simulink model "LATC_Test_Calc"  (R2021b)
settings: Solver=FixedStepDiscrete  StartTime=0.0  StopTime=inf  FixedStep=0.01  RelTol=1e-3
undefined symbols (not defined in the file or in its folder): P_LCS_A0_Dis_BP, P_LCS_A2_Curve_BP, P_LCS_A2S_FliterTime, P_LCS_DeltaEps_SpdBp, P_LCS_LCC_A0_Dis_BP, P_LCS_LCC_AngleSlope_ELK, P_LCS_LCC_AngleSlope_ESS, P_LCS_LCC_AngleSlope_LCCancle, P_LCS_LCC_AngleSlope_LCEco, P_LCS_LCC_AngleSlope_LCK, P_LCS_LCC_AngleSlope_LCKIE, P_LCS_LCC_AngleSlope_LCNomal, P_LCS_LCC_AngleSlope_LCSport, P_LCS_LCC_AngleSlope_LKA, P_LCS_LCC_Eco_AyDtLimit_TBL, P_LCS_LCC_ELK_AyDtLimit_TBL, P_LCS_LCC_ESS_AyDtLimit_TBL, P_LCS_LCC_LC_AyDtLimit_TBL, P_LCS_LCC_LC_Normal_AyDtLimit_TBL, P_LCS_LCC_LC_Planning_Dist_TBL, P_LCS_LCC_LCK_AyDtLimit_TBL, P_LCS_LCC_LCK_Planning_Dist_TBL, P_LCS_LCC_LKA_AyDtLimit_TBL, P_LCS_LCC_Matrix_q1_st, P_LCS_LCC_Matrix_q2_st, P_LCS_LCC_Max_Lateral_Acc_ms2, P_LCS_LCC_MaxLatAcc_ELK, P_LCS_LCC_MaxLatAcc_ESS, P_LCS_LCC_MaxLatAcc_LCCancel, P_LCS_LCC_MaxLatAcc_LCEco, P_LCS_LCC_MaxLatAcc_LCK, P_LCS_LCC_MaxLatAcc_LCKIE, P_LCS_LCC_MaxLatAcc_LCNomal, P_LCS_LCC_MaxLatAcc_LCSport, P_LCS_LCC_MaxLatAcc_LKA, P_LCS_LCC_Min_Plan_Dis, P_LCS_LCC_PlaningLength_m, P_LCS_LCC_PreCur_Min_Plan_Dis_Fac, P_LCS_LCC_PreView_Fac, P_LCS_LCC_PreView_s, P_LCS_LCC_PreViewCurve_Fac, P_LCS_LCC_PreViewT, P_LCS_LCC_Spd_BP, P_LCS_LCC_Spd_BP2, P_LCS_LCC_Sport_AyDtLimit_TBL, P_LCS_LCC_StateActiv_AyDtLimit, P_LCS_LCC_StateActiv_PreviewT, P_LCS_LCC_StateActiveDelaytime, P_LCS_LCC_TarSteerAngleSlope, P_LCS_preDis_spd, P_LCS_StateActiv_AngleSlope, P_LCS_StateActive_HoldTime_BP, P_LCS_StateActiveFlg_BP, P_LCS_StateHold_time
libraries: canapelib x35, simulink x2
(part 1 of 3)
settings Model: DataDictionary=HWAtest.sldd  Creator=GW00216231  LastModifiedBy=GW00201118
settings SolverCC: AlgebraicLoopSolver=TrustRegion
settings OptimizationCC: DefaultParameterBehavior=Inlined  EnhancedBackFolding=on  PassReuseOutputArgsThreshold=0  OptimizeBlockOrder=speed  DifferentSizesBufferReuse=on  OptimizationCustomize=off
settings DebuggingCC: SignalResolutionControl=TryResolveAllWithWarning  ParameterTunabilityLossMsg=error  SFMachineParentedDataDiag=warning  UnderSpecifiedDimensionMsg=warning
settings SFSimCC: MATLABDynamicMemAlloc=off
settings RTWCC: Description=Vector CANape/vSignalyzer Target (Visual C/C++ Project Makefile)  SystemTargetFile=cnp.tlc  TemplateMakefile=cnp_msdll.tmf
settings CodeAppCC: ForceParamTrailComments=on  OperatorAnnotations=on
settings STFCustomTargetCC: MATLABClassNameForMDSCustomization=Simulink.SoftwareTarget.TargetSpecificTriggerConfigurationBase  SystemTargetFile=cnp.tlc

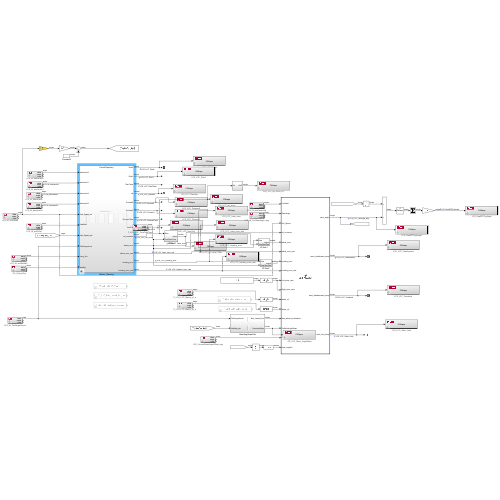
[thumbnail: Simulink's stored preview of the top-level diagram]
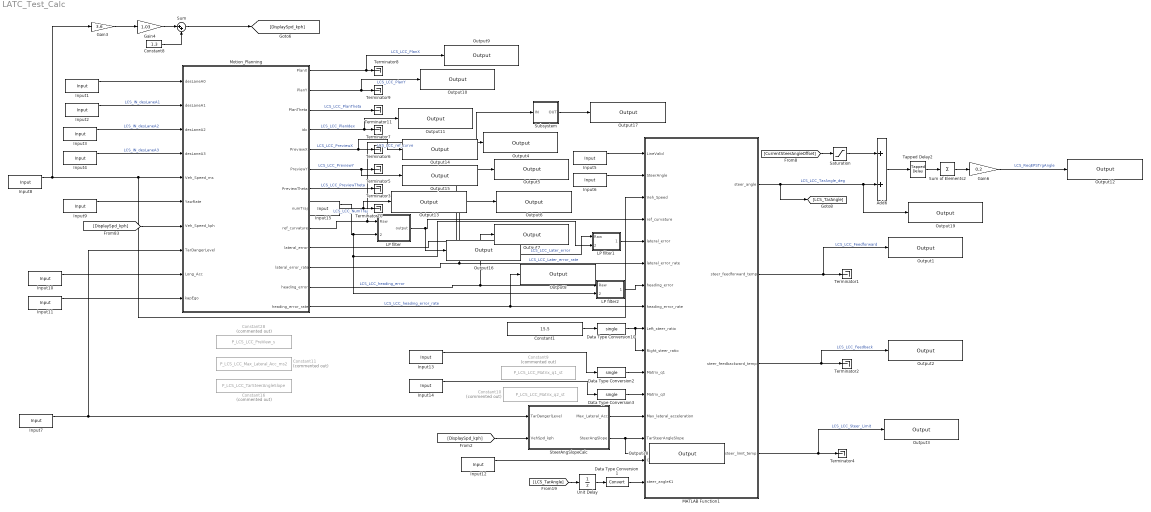
== system LATC_Test_Calc ==
  Add6 : Sum  AccumDataTypeStr=single
  Constant1 : Constant  Value=15.5  OutDataTypeStr=single
  Constant10 : Constant  Commented=on  Value=P_LCS_LCC_Matrix_q2_st  OutDataTypeStr=single
  Constant11 : Constant  Commented=on  Value=P_LCS_LCC_Max_Lateral_Acc_ms2  OutDataTypeStr=single
  Constant16 : Constant  Commented=on  Value=P_LCS_LCC_TarSteerAngleSlope  OutDataTypeStr=single
  Constant28 : Constant  Commented=on  Value=P_LCS_LCC_PreView_s  OutDataTypeStr=single
  Constant8 : Constant  Value=1.3  OutDataTypeStr=single
  Constant9 : Constant  Commented=on  Value=P_LCS_LCC_Matrix_q1_st  OutDataTypeStr=single
  Data Type Conversion1 : DataTypeConversion
  Data Type Conversion10 : DataTypeConversion  OutDataTypeStr=single
  Data Type Conversion2 : DataTypeConversion  OutDataTypeStr=single
  Data Type Conversion3 : DataTypeConversion  OutDataTypeStr=single
  Gain3 : Gain  Gain=3.6
  Gain4 : Gain  Gain=1.03
  Gain6 : Gain  Gain=0.2
  Input1 : canapelib/CANape I//O/Input  envName=LCS_IN_desLaneA0  envRows=1  envCols=1  envDataType=float  swInheritSampleTime=on  envPortId=0
      settings: AttributesFormatString=%<envName>  SourceProductName=Vector CANape/vSignalyzer Target
  Input10 : canapelib/CANape I//O/Input  envName=LCS_IN_axvRefMs2  envRows=1  envCols=1  envDataType=float  swInheritSampleTime=on  envPortId=0
      settings: AttributesFormatString=%<envName>  SourceProductName=Vector CANape/vSignalyzer Target
  Input11 : canapelib/CANape I//O/Input  envName=LCS_IN_kapTraj  envRows=1  envCols=1  envDataType=float  swInheritSampleTime=on  envPortId=0
      settings: AttributesFormatString=%<envName>  SourceProductName=Vector CANape/vSignalyzer Target
  Input12 : canapelib/CANape I//O/Input  envName=LCS_CurrentSteerAngleOffset_deg  envRows=1  envCols=1  envDataType=float  swInheritSampleTime=on  envPortId=0
      settings: AttributesFormatString=%<envName>  SourceProductName=Vector CANape/vSignalyzer Target
  Input13 : canapelib/CANape I//O/Input  envName=P_LCS_LCC_Matrix_q1_st  envRows=1  envCols=1  envDataType=float  swInheritSampleTime=on  envPortId=0
      settings: AttributesFormatString=%<envName>  SourceProductName=Vector CANape/vSignalyzer Target
  Input14 : canapelib/CANape I//O/Input  envName=P_LCS_LCC_Matrix_q2_st  envRows=1  envCols=1  envDataType=float  swInheritSampleTime=on  envPortId=0
      settings: AttributesFormatString=%<envName>  SourceProductName=Vector CANape/vSignalyzer Target
  Input15 : canapelib/CANape I//O/Input  envName=P_LCS_LCC_CureFilterTime  envRows=1  envCols=1  envDataType=float  swInheritSampleTime=on  envPortId=0
      settings: AttributesFormatString=%<envName>  SourceProductName=Vector CANape/vSignalyzer Target
  Input2 : canapelib/CANape I//O/Input  envName=LCS_IN_desLaneA1  envRows=1  envCols=1  envDataType=float  swInheritSampleTime=on  envPortId=0
      settings: AttributesFormatString=%<envName>  SourceProductName=Vector CANape/vSignalyzer Target
  Input3 : canapelib/CANape I//O/Input  envName=LCS_IN_desLaneA2  envRows=1  envCols=1  envDataType=float  swInheritSampleTime=on  envPortId=0
      settings: AttributesFormatString=%<envName>  SourceProductName=Vector CANape/vSignalyzer Target
  Input4 : canapelib/CANape I//O/Input  envName=LCS_IN_desLaneA3  envRows=1  envCols=1  envDataType=float  swInheritSampleTime=on  envPortId=0
      settings: AttributesFormatString=%<envName>  SourceProductName=Vector CANape/vSignalyzer Target
  Input5 : canapelib/CANape I//O/Input  envName=LCS_IN_desLaneValid  envRows=1  envCols=1  envDataType=float  swInheritSampleTime=on  envPortId=0
      settings: AttributesFormatString=%<envName>  SourceProductName=Vector CANape/vSignalyzer Target
  Input6 : canapelib/CANape I//O/Input  envName=LCS_IN_CurSteerAngle_deg  envRows=1  envCols=1  envDataType=float  swInheritSampleTime=on  envPortId=0
      settings: AttributesFormatString=%<envName>  SourceProductName=Vector CANape/vSignalyzer Target
  Input7 : canapelib/CANape I//O/Input  envName=LCS_IN_TarDangerlLevel  envRows=1  envCols=1  envDataType=uint8  swInheritSampleTime=on  envPortId=0
      settings: AttributesFormatString=%<envName>  SourceProductName=Vector CANape/vSignalyzer Target
  Input8 : canapelib/CANape I//O/Input  envName=LCS_IN_vxvRefMs  envRows=1  envCols=1  envDataType=float  swInheritSampleTime=on  envPortId=0
      settings: AttributesFormatString=%<envName>  SourceProductName=Vector CANape/vSignalyzer Target
  Input9 : canapelib/CANape I//O/Input  envName=LCS_IN_psiDtOpt  envRows=1  envCols=1  envDataType=float  swInheritSampleTime=on  envPortId=0
      settings: AttributesFormatString=%<envName>  SourceProductName=Vector CANape/vSignalyzer Target
  LP filter : Subsystem
  LP filter1 : Subsystem
  LP filter2 : Subsystem
  MATLAB Function1 : MATLAB Function  TreatAsAtomicUnit=on
  Motion_Planning : Subsystem  Variant=on  VariantControlMode=label  LabelModeActiveChoice=Choice_3
  Output1 : canapelib/CANape I//O/Output  envName=LCS_LCC_Feedforward  envRows=1  envCols=1  envPortId=0
      settings: AttributesFormatString=%<envName>  SourceProductName=Vector CANape/vSignalyzer Target
  Output10 : canapelib/CANape I//O/Output  envName=LCS_LCC_PlanY  envRows=40  envCols=1  envPortId=0
      settings: AttributesFormatString=%<envName>  SourceProductName=Vector CANape/vSignalyzer Target
  Output11 : canapelib/CANape I//O/Output  envName=LCS_LCC_PlanIdex  envRows=1  envCols=1  envPortId=0
      settings: AttributesFormatString=%<envName>  SourceProductName=Vector CANape/vSignalyzer Target
  Output12 : canapelib/CANape I//O/Output  envName=LCS_ReqEPSTrgAngle  envRows=1  envCols=1  envPortId=0
      settings: AttributesFormatString=%<envName>  SourceProductName=Vector CANape/vSignalyzer Target
  Output13 : canapelib/CANape I//O/Output  envName=LCS_LCC_NumTraj  envRows=1  envCols=1  envPortId=0
      settings: AttributesFormatString=%<envName>  SourceProductName=Vector CANape/vSignalyzer Target
  Output14 : canapelib/CANape I//O/Output  envName=LCS_LCC_PreviewX  envRows=1  envCols=1  envPortId=0
      settings: AttributesFormatString=%<envName>  SourceProductName=Vector CANape/vSignalyzer Target
  Output15 : canapelib/CANape I//O/Output  envName=LCS_LCC_PreviewY  envRows=1  envCols=1  envPortId=0
      settings: AttributesFormatString=%<envName>  SourceProductName=Vector CANape/vSignalyzer Target
  Output16 : canapelib/CANape I//O/Output  envName=LCS_LCC_ref_curve_Filter  envRows=1  envCols=1  envPortId=0
      settings: AttributesFormatString=%<envName>  SourceProductName=Vector CANape/vSignalyzer Target
  Output17 : canapelib/CANape I//O/Output  envName=LCS_LCC_ref_curve_Av  envRows=1  envCols=1  envPortId=0
      settings: AttributesFormatString=%<envName>  SourceProductName=Vector CANape/vSignalyzer Target
  Output18 : canapelib/CANape I//O/Output  envName=LCS_LCC_Steer_AngleSlope  envRows=1  envCols=1  envPortId=0
      settings: AttributesFormatString=%<envName>  SourceProductName=Vector CANape/vSignalyzer Target
  Output19 : canapelib/CANape I//O/Output  envName=LCS_ReqEPSTrgAngle1  envRows=1  envCols=1  envPortId=0
      settings: AttributesFormatString=%<envName>  SourceProductName=Vector CANape/vSignalyzer Target
  Output2 : canapelib/CANape I//O/Output  envName=LCS_LCC_Feedback  envRows=1  envCols=1  envPortId=0
      settings: AttributesFormatString=%<envName>  SourceProductName=Vector CANape/vSignalyzer Target
  Output3 : canapelib/CANape I//O/Output  envName=LCS_LCC_Steer_Limit  envRows=1  envCols=1  envPortId=0
      settings: AttributesFormatString=%<envName>  SourceProductName=Vector CANape/vSignalyzer Target
  Output4 : canapelib/CANape I//O/Output  envName=LCS_LCC_ref_curve  envRows=1  envCols=1  envPortId=0
      settings: AttributesFormatString=%<envName>  SourceProductName=Vector CANape/vSignalyzer Target
  Output5 : canapelib/CANape I//O/Output  envName=LCS_LCC_Later_error  envRows=1  envCols=1  envPortId=0
      settings: AttributesFormatString=%<envName>  SourceProductName=Vector CANape/vSignalyzer Target
  Output6 : canapelib/CANape I//O/Output  envName=LCS_LCC_Later_error_rate  envRows=1  envCols=1  envPortId=0
      settings: AttributesFormatString=%<envName>  SourceProductName=Vector CANape/vSignalyzer Target
  Output7 : canapelib/CANape I//O/Output  envName=LCS_LCC_heading_error  envRows=1  envCols=1  envPortId=0
      settings: AttributesFormatString=%<envName>  SourceProductName=Vector CANape/vSignalyzer Target
  Output8 : canapelib/CANape I//O/Output  envName=LCS_LCC_heading_error_rate  envRows=1  envCols=1  envPortId=0
      settings: AttributesFormatString=%<envName>  SourceProductName=Vector CANape/vSignalyzer Target
  Output9 : canapelib/CANape I//O/Output  envName=LCS_LCC_PlanX  envRows=40  envCols=1  envPortId=0
      settings: AttributesFormatString=%<envName>  SourceProductName=Vector CANape/vSignalyzer Target
  Saturation : Saturate  UpperLimit=10  LowerLimit=-10  OutDataTypeStr=single
  SteerAngSlopeCalc : Subsystem
  Subsystem : Subsystem
  Sum : Sum  Inputs=|++
  Sum of Elements2 : Sum  Inputs=+
  Tapped Delay2 : simulink/Discrete/Tapped Delay  vinit=0.0  samptime=-1  NumDelays=4  DelayOrder=Newest  includeCurrent=on
  Terminator{1..11} (11 alike) : Terminator
  Unit Delay : UnitDelay  SampleTime=-1  HasFrameUpgradeWarning=on
  wires:
  [DisplaySpd_kph] -> Motion_Planning/7(Veh_Speed_kph)
  Input10/1 -> Motion_Planning/9(Long_Acc)
  Sum of Elements2/1 -> Gain6/1
  Motion_Planning/11(lateral_error_rate) -> Output6/1, MATLAB Function1/6(lateral_error_rate)  "LCS_LCC_Later_error_rate"
  Input8/1 -> Gain3/1, MATLAB Function1/3(Veh_Speed), Motion_Planning/5(Veh_Speed_ms)
  MATLAB Function1/2(steer_feedforward_temp) -> Output1/1, Terminator1/1  "LCS_LCC_Feedforward"
  Input12/1 -> MATLAB Function1/15(CurrentSteerAngleOffset)
  Gain6/1 -> Output12/1  "LCS_ReqEPSTrgAngle"
  MATLAB Function1/4(steer_limit_temp) -> Output3/1, Terminator4/1  "LCS_LCC_Steer_Limit"
  SteerAngSlopeCalc/1(Max_Lateral_Acc) -> MATLAB Function1/13(Max_lateral_acceleration)
  Add6/1 -> Tapped Delay2/1
  SteerAngSlopeCalc/2(SteerAngSlope) -> Output18/1, MATLAB Function1/14(TarSteerAngleSlope)
  [LCS_TarAngle] -> Unit Delay/1
  MATLAB Function1/3(steer_feedbackward_temp) -> Output2/1, Terminator2/1  "LCS_LCC_Feedback"
  Motion_Planning/4(idx) -> Output11/1, Terminator7/1  "LCS_LCC_PlanIdex"
  [DisplaySpd_kph] -> SteerAngSlopeCalc/2(VehSpd_kph)
  LP filter/1(output) -> Output16/1, MATLAB Function1/4(ref_curvature)
  Data Type Conversion2/1 -> MATLAB Function1/11(Matrix_q1)
  Motion_Planning/10(lateral_error) -> LP filter1/1(Raw), Output5/1  "LCS_LCC_Later_error"
  Motion_Planning/2(PlanY) -> Output10/1, Terminator9/1  "LCS_LCC_PlanY"
  Motion_Planning/6(PreviewY) -> Output15/1, Terminator5/1  "LCS_LCC_PreviewY"
  Input5/1 -> MATLAB Function1/1(LineValid)
  Input1/1 -> Motion_Planning/1(desLaneA0)
  Saturation/1 -> Add6/1
  Input6/1 -> MATLAB Function1/2(SteerAngle)
  Motion_Planning/3(PlanTheta) -> Terminator11/1  "LCS_LCC_PlanTheta"
  Motion_Planning/12(heading_error) -> Output7/1, LP filter2/1(Raw)  "LCS_LCC_heading_error"
  Unit Delay/1 -> Data Type Conversion1/1
  Input2/1 -> Motion_Planning/2(desLaneA1)  "LCS_IN_desLaneA1"
  Input11/1 -> Motion_Planning/10(kapEgo)
  Data Type Conversion10/1 -> MATLAB Function1/10(Right_steer_ratio), MATLAB Function1/9(Left_steer_ratio)
  Input14/1 -> Data Type Conversion3/1
  Input4/1 -> Motion_Planning/4(desLaneA3)  "LCS_IN_desLaneA3"
  Motion_Planning/7(PreviewTheta) -> Terminator3/1  "LCS_LCC_PreviewTheta"
  Input7/1 -> Motion_Planning/8(TarDangerLevel), SteerAngSlopeCalc/1(TarDangerlLevel)
  Motion_Planning/13(heading_error_rate) -> Output8/1, MATLAB Function1/8(heading_error_rate)  "LCS_LCC_heading_error_rate"
  Tapped Delay2/1 -> Sum of Elements2/1
  Input9/1 -> Motion_Planning/6(YawRate)
  Input3/1 -> Motion_Planning/3(desLaneA2)  "LCS_IN_desLaneA2"
  Data Type Conversion1/1 -> MATLAB Function1/16(steer_angleK1)
  [CurrentSteerAngleOffset] -> Saturation/1
  MATLAB Function1/1(steer_angle) -> [LCS_TarAngle], Output19/1, Add6/2  "LCS_LCC_TarAngle_deg"
  Motion_Planning/1(PlanX) -> Output9/1, Terminator8/1  "LCS_LCC_PlanX"
  Constant1/1 -> Data Type Conversion10/1
  Motion_Planning/5(PreviewX) -> Output14/1, Terminator6/1  "LCS_LCC_PreviewX"
  Data Type Conversion3/1 -> MATLAB Function1/12(Matrix_q3)
  Motion_Planning/8(numTraj) -> Output13/1, Terminator10/1  "LCS_LCC_NumTraj"
  Input13/1 -> Data Type Conversion2/1
  Sum/1 -> [DisplaySpd_kph]
  Gain3/1 -> Gain4/1
  Gain4/1 -> Sum/1
  Constant8/1 -> Sum/2
  Motion_Planning/9(ref_curvature) -> Subsystem/1(IN), Output4/1, LP filter/1(Raw)  "LCS_LCC_ref_curve"
  Subsystem/1(OUT) -> Output17/1
  LP filter1/1(output) -> MATLAB Function1/5(lateral_error)
  LP filter2/1(output) -> MATLAB Function1/7(heading_error)
  Input15/1 -> LP filter2/2(TorqFilterTime), LP filter1/2(TorqFilterTime), LP filter/2(TorqFilterTime)

== system LATC_Test_Calc/LP filter ==
  Raw : Inport
  TorqFilterTime : Inport  Port=2
  Memory2 : Memory  InheritSampleTime=on
  Product1 : Product  RndMeth=Zero
  Product4 : Product  Inputs=*/  RndMeth=Zero
  Sum4 : Sum  Inputs=+-|
  Sum5 : Sum  Inputs=++|
  Weight/N3 : Constant  Value=0.02  OutDataTypeStr=single
  output : Outport
  wires:
  TorqFilterTime/1 -> Product4/2
  Product4/1 -> Product1/1
  Weight/N3/1 -> Product4/1
  Raw/1 -> Sum4/1
  Product1/1 -> Sum5/1
  Sum4/1 -> Product1/2
  Memory2/1 -> Sum4/2, Sum5/2
  Sum5/1 -> output/1, Memory2/1

== system LATC_Test_Calc/LP filter1 ==
  Raw : Inport
  TorqFilterTime : Inport  Port=2
  Memory2 : Memory  InheritSampleTime=on
  Product1 : Product  RndMeth=Zero
  Product4 : Product  Inputs=*/  RndMeth=Zero
  Sum4 : Sum  Inputs=+-|
  Sum5 : Sum  Inputs=++|
  Weight/N3 : Constant  Value=0.02  OutDataTypeStr=single
  output : Outport
  wires:
  Sum5/1 -> Memory2/1, output/1
  Memory2/1 -> Sum5/2, Sum4/2
  Sum4/1 -> Product1/2
  Product1/1 -> Sum5/1
  Raw/1 -> Sum4/1
  Weight/N3/1 -> Product4/1
  Product4/1 -> Product1/1
  TorqFilterTime/1 -> Product4/2

== system LATC_Test_Calc/LP filter2 ==
  Raw : Inport
  TorqFilterTime : Inport  Port=2
  Memory2 : Memory  InheritSampleTime=on
  Product1 : Product  RndMeth=Zero
  Product4 : Product  Inputs=*/  RndMeth=Zero
  Sum4 : Sum  Inputs=+-|
  Sum5 : Sum  Inputs=++|
  Weight/N3 : Constant  Value=0.02  OutDataTypeStr=single
  output : Outport
  wires:
  TorqFilterTime/1 -> Product4/2
  Product4/1 -> Product1/1
  Weight/N3/1 -> Product4/1
  Raw/1 -> Sum4/1
  Product1/1 -> Sum5/1
  Sum4/1 -> Product1/2
  Memory2/1 -> Sum4/2, Sum5/2
  Sum5/1 -> output/1, Memory2/1

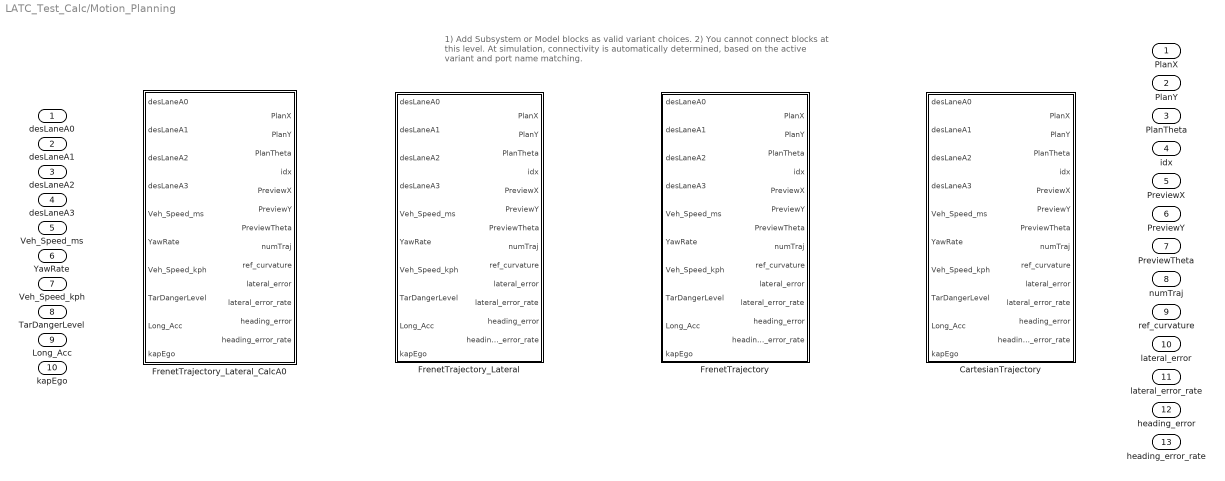
== system LATC_Test_Calc/Motion_Planning ==
  note: 1) Add Subsystem or Model blocks as valid variant choices.
      | 2) You cannot connect blocks at this level. At simulation, connectivity is automatically
      | determined, based on the active variant and port name matching.
  desLaneA0 : Inport
  desLaneA1 : Inport  Port=2
  desLaneA2 : Inport  Port=3
  desLaneA3 : Inport  Port=4
  Veh_Speed_ms : Inport  Port=5
  YawRate : Inport  Port=6
  Veh_Speed_kph : Inport  Port=7
  TarDangerLevel : Inport  Port=8
  Long_Acc : Inport  Port=9
  kapEgo : Inport  Port=10
  CartesianTrajectory : Subsystem  VariantControl=Choice_4
  FrenetTrajectory : Subsystem  VariantControl=Choice_3
  FrenetTrajectory_Lateral : Subsystem  VariantControl=Choice_2
  FrenetTrajectory_Lateral_CalcA0 : Subsystem  VariantControl=Choice_1
  PlanX : Outport
  PlanY : Outport  Port=2
  PlanTheta : Outport  Port=3
  idx : Outport  Port=4
  PreviewX : Outport  Port=5
  PreviewY : Outport  Port=6
  PreviewTheta : Outport  Port=7
  numTraj : Outport  Port=8
  ref_curvature : Outport  Port=9
  lateral_error : Outport  Port=10
  lateral_error_rate : Outport  Port=11
  heading_error : Outport  Port=12
  heading_error_rate : Outport  Port=13

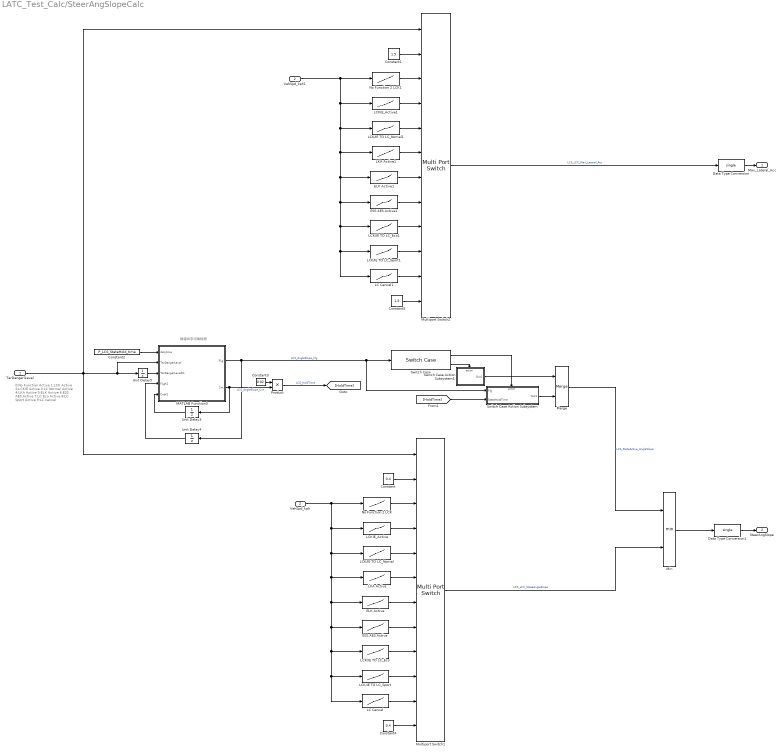
== system LATC_Test_Calc/SteerAngSlopeCalc ==
  note: 0:No Function Active
      | 1:LCK Active
      | 2:LCKIE Active
      | 3:LC Normal Active
      | 4:LKA Active
      | 5:ELK Active
      | 6:ESS AES Active
      | 7:LC Eco Active
      | 8:LC Sport Active
      | 9:LC cancel
  note: 换道状态切换检测
  TarDangerlLevel : Inport
  VehSpd_kph : Inport  Port=2
  Constant : Constant  Value=0.4  OutDataTypeStr=single
  Constant1 : Constant  Value=1.5  OutDataTypeStr=single
  Constant2 : Constant  Value=P_LCS_StateHold_time  OutDataTypeStr=uint16
  Constant3 : Constant  Value=0.02
  Constant4 : Constant  Value=0.4  OutDataTypeStr=single
  Constant5 : Constant  Value=1.5  OutDataTypeStr=single
  Data Type Conversion : DataTypeConversion  OutDataTypeStr=single
  Data Type Conversion1 : DataTypeConversion  OutDataTypeStr=single
  ELK Active : Lookup_n-D  NumberOfTableDimensions=1  BreakpointsForDimension1=P_LCS_preDis_spd  Table=P_LCS_LCC_AngleSlope_ELK  ExtrapMethod=Clip  InternalRulePriority=Speed  RndMeth=Simplest  InputSameDT=on
  ELK Active1 : Lookup_n-D  NumberOfTableDimensions=1  BreakpointsForDimension1=P_LCS_preDis_spd  Table=P_LCS_LCC_MaxLatAcc_ELK  ExtrapMethod=Clip  InternalRulePriority=Speed  RndMeth=Simplest  InputSameDT=on
  ESS AES Active : Lookup_n-D  NumberOfTableDimensions=1  BreakpointsForDimension1=P_LCS_preDis_spd  Table=P_LCS_LCC_AngleSlope_ESS  ExtrapMethod=Clip  InternalRulePriority=Speed  RndMeth=Simplest  InputSameDT=on
  ESS AES Active1 : Lookup_n-D  NumberOfTableDimensions=1  BreakpointsForDimension1=P_LCS_preDis_spd  Table=P_LCS_LCC_MaxLatAcc_ESS  ExtrapMethod=Clip  InternalRulePriority=Speed  RndMeth=Simplest  InputSameDT=on
  LC Cancel : Lookup_n-D  NumberOfTableDimensions=1  BreakpointsForDimension1=P_LCS_preDis_spd  Table=P_LCS_LCC_AngleSlope_LCCancle  ExtrapMethod=Clip  InternalRulePriority=Speed  RndMeth=Simplest  InputSameDT=on
  LC Cancel1 : Lookup_n-D  NumberOfTableDimensions=1  BreakpointsForDimension1=P_LCS_preDis_spd  Table=P_LCS_LCC_MaxLatAcc_LCCancel  ExtrapMethod=Clip  InternalRulePriority=Speed  RndMeth=Simplest  InputSameDT=on
  LCK/IE TO LC_Eco : Lookup_n-D  NumberOfTableDimensions=1  BreakpointsForDimension1=P_LCS_preDis_spd  Table=P_LCS_LCC_AngleSlope_LCEco  ExtrapMethod=Clip  InternalRulePriority=Speed  RndMeth=Simplest  InputSameDT=on
  LCK/IE TO LC_Eco1 : Lookup_n-D  NumberOfTableDimensions=1  BreakpointsForDimension1=P_LCS_preDis_spd  Table=P_LCS_LCC_MaxLatAcc_LCEco  ExtrapMethod=Clip  InternalRulePriority=Speed  RndMeth=Simplest  InputSameDT=on
  LCK/IE TO LC_Nomal : Lookup_n-D  NumberOfTableDimensions=1  BreakpointsForDimension1=P_LCS_preDis_spd  Table=P_LCS_LCC_AngleSlope_LCNomal  ExtrapMethod=Clip  InternalRulePriority=Speed  RndMeth=Simplest  InputSameDT=on
  LCK/IE TO LC_Nomal1 : Lookup_n-D  NumberOfTableDimensions=1  BreakpointsForDimension1=P_LCS_preDis_spd  Table=P_LCS_LCC_MaxLatAcc_LCNomal  ExtrapMethod=Clip  InternalRulePriority=Speed  RndMeth=Simplest  InputSameDT=on
  LCK/IE TO LC_Sport : Lookup_n-D  NumberOfTableDimensions=1  BreakpointsForDimension1=P_LCS_preDis_spd  Table=P_LCS_LCC_AngleSlope_LCSport  ExtrapMethod=Clip  InternalRulePriority=Speed  RndMeth=Simplest  InputSameDT=on
  LCK/IE TO LC_Sport1 : Lookup_n-D  NumberOfTableDimensions=1  BreakpointsForDimension1=P_LCS_preDis_spd  Table=P_LCS_LCC_MaxLatAcc_LCSport  ExtrapMethod=Clip  InternalRulePriority=Speed  RndMeth=Simplest  InputSameDT=on
  LCKIE_Active : Lookup_n-D  NumberOfTableDimensions=1  BreakpointsForDimension1=P_LCS_preDis_spd  Table=P_LCS_LCC_AngleSlope_LCKIE  ExtrapMethod=Clip  InternalRulePriority=Speed  RndMeth=Simplest  InputSameDT=on
  LCKIE_Active1 : Lookup_n-D  NumberOfTableDimensions=1  BreakpointsForDimension1=P_LCS_preDis_spd  Table=P_LCS_LCC_MaxLatAcc_LCKIE  ExtrapMethod=Clip  InternalRulePriority=Speed  RndMeth=Simplest  InputSameDT=on
  LKA Active : Lookup_n-D  NumberOfTableDimensions=1  BreakpointsForDimension1=P_LCS_preDis_spd  Table=P_LCS_LCC_AngleSlope_LKA  ExtrapMethod=Clip  InternalRulePriority=Speed  RndMeth=Simplest  InputSameDT=on
  LKA Active1 : Lookup_n-D  NumberOfTableDimensions=1  BreakpointsForDimension1=P_LCS_preDis_spd  Table=P_LCS_LCC_MaxLatAcc_LKA  ExtrapMethod=Clip  InternalRulePriority=Speed  RndMeth=Simplest  InputSameDT=on
  MATLAB Function3 : MATLAB Function  TreatAsAtomicUnit=on
  Merge : Merge
  Min : MinMax  Inputs=2
  Multiport Switch1 : MultiPortSwitch  DataPortOrder=Zero-based contiguous  Inputs=11  zeroidx=on
  Multiport Switch2 : MultiPortSwitch  DataPortOrder=Zero-based contiguous  Inputs=11  zeroidx=on
  No Function 2 LCK : Lookup_n-D  NumberOfTableDimensions=1  BreakpointsForDimension1=P_LCS_preDis_spd  Table=P_LCS_LCC_AngleSlope_LCK  ExtrapMethod=Clip  InternalRulePriority=Speed  RndMeth=Simplest  InputSameDT=on
  No Function 2 LCK1 : Lookup_n-D  NumberOfTableDimensions=1  BreakpointsForDimension1=P_LCS_preDis_spd  Table=P_LCS_LCC_MaxLatAcc_LCK  ExtrapMethod=Clip  InternalRulePriority=Speed  RndMeth=Simplest  InputSameDT=on
  Product : Product
  Switch Case : SwitchCase  CaseConditions={[1,2,3,4,5]}
  Switch Case Action Subsystem : Subsystem  TreatAsAtomicUnit=on
  Switch Case Action Subsystem1 : Subsystem  TreatAsAtomicUnit=on
  Unit Delay3 : UnitDelay  SampleTime=-1  HasFrameUpgradeWarning=on
  Unit Delay4 : UnitDelay  SampleTime=-1  HasFrameUpgradeWarning=on
  Unit Delay5 : UnitDelay  SampleTime=-1  HasFrameUpgradeWarning=on
  VehSpd_kph1 : InportShadow  Port=2
  Max_Lateral_Acc : Outport  OutDataTypeStr=single
  SteerAngSlope : Outport  Port=2  OutDataTypeStr=single
  wires:
  TarDangerlLevel/1 -> Multiport Switch1/1, Multiport Switch2/1, Unit Delay5/1, MATLAB Function3/2(TarDangerLevel)
  Merge/1 -> Min/1  "LCS_StateActive_AngleSlope"
  Switch Case Action Subsystem1/1(Out1) -> Merge/1
  Switch Case Action Subsystem/1(Out1) -> Merge/2
  [HoldTime] -> Switch Case Action Subsystem/2(StateHoldTime)
  Switch Case/2 -> Switch Case Action Subsystem1/Action
  Switch Case/1 -> Switch Case Action Subsystem/Action
  LCK/IE TO LC_Nomal/1 -> Multiport Switch1/5
  Min/1 -> Data Type Conversion1/1
  Product/1 -> [HoldTime]  "LCS_HoldTime"
  Constant3/1 -> Product/1
  Constant4/1 -> Multiport Switch1/12
  LKA Active/1 -> Multiport Switch1/6
  No Function 2 LCK/1 -> Multiport Switch1/3
  Multiport Switch1/1 -> Min/2  "LCS_LCC_StateAngleSlope"
  Constant2/1 -> MATLAB Function3/1(delytime)
  MATLAB Function3/1(FLg) -> Unit Delay4/1, Switch Case Action Subsystem/1(Flg), Switch Case/1  "LCS_AngleSlope_Flg"
  MATLAB Function3/2(Cnt) -> Unit Delay3/1, Product/2  "LCS_AngleSlope_Cnt"
  Constant/1 -> Multiport Switch1/2
  Unit Delay4/1 -> MATLAB Function3/4(FLgK1)
  Unit Delay3/1 -> MATLAB Function3/5(CntK1)
  LCKIE_Active/1 -> Multiport Switch1/4
  ELK Active/1 -> Multiport Switch1/7
  VehSpd_kph/1 -> No Function 2 LCK/1, LCK/IE TO LC_Nomal/1, LC Cancel/1, LCK/IE TO LC_Sport/1, LCK/IE TO LC_Eco/1, ESS AES Active/1, ELK Active/1, LKA Active/1, LCKIE_Active/1
  Unit Delay5/1 -> MATLAB Function3/3(TarDangerLevelK1)
  ESS AES Active/1 -> Multiport Switch1/8
  LCK/IE TO LC_Eco/1 -> Multiport Switch1/9
  LCK/IE TO LC_Sport/1 -> Multiport Switch1/10
  LC Cancel/1 -> Multiport Switch1/11
  Multiport Switch2/1 -> Data Type Conversion/1  "LCS_LCC_Max_Lateral_Acc"
  Constant1/1 -> Multiport Switch2/2
  Constant5/1 -> Multiport Switch2/12
  LC Cancel1/1 -> Multiport Switch2/11
  LCK/IE TO LC_Sport1/1 -> Multiport Switch2/10
  LCK/IE TO LC_Eco1/1 -> Multiport Switch2/9
  ESS AES Active1/1 -> Multiport Switch2/8
  VehSpd_kph1/1 -> LCKIE_Active1/1, LKA Active1/1, ELK Active1/1, ESS AES Active1/1, LCK/IE TO LC_Eco1/1, LCK/IE TO LC_Sport1/1, LC Cancel1/1, LCK/IE TO LC_Nomal1/1, No Function 2 LCK1/1
  ELK Active1/1 -> Multiport Switch2/7
  LCKIE_Active1/1 -> Multiport Switch2/4
  No Function 2 LCK1/1 -> Multiport Switch2/3
  LKA Active1/1 -> Multiport Switch2/6
  LCK/IE TO LC_Nomal1/1 -> Multiport Switch2/5
  Data Type Conversion/1 -> Max_Lateral_Acc/1
  Data Type Conversion1/1 -> SteerAngSlope/1

== system LATC_Test_Calc/Subsystem ==
  IN : Inport
  Gain1 : Gain  Gain=0.2
  Sum of Elements1 : Sum  Inputs=+
  Tapped Delay1 : simulink/Discrete/Tapped Delay  vinit=0.0  samptime=-1  NumDelays=4  DelayOrder=Newest  includeCurrent=on
  OUT : Outport
  wires:
  IN/1 -> Tapped Delay1/1
  Tapped Delay1/1 -> Sum of Elements1/1
  Sum of Elements1/1 -> Gain1/1
  Gain1/1 -> OUT/1

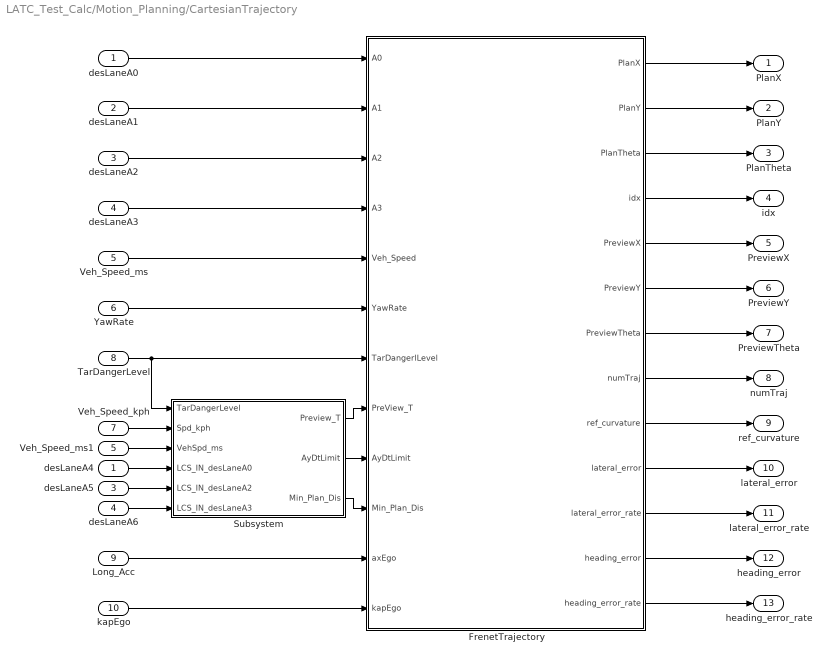
== system LATC_Test_Calc/Motion_Planning/CartesianTrajectory ==
  desLaneA0 : Inport
  desLaneA1 : Inport  Port=2
  desLaneA2 : Inport  Port=3
  desLaneA3 : Inport  Port=4
  Veh_Speed_ms : Inport  Port=5
  YawRate : Inport  Port=6
  Veh_Speed_kph : Inport  Port=7
  TarDangerLevel : Inport  Port=8
  Long_Acc : Inport  Port=9
  kapEgo : Inport  Port=10
  FrenetTrajectory : MATLAB Function  TreatAsAtomicUnit=on
  Subsystem : Subsystem
  Veh_Speed_ms1 : InportShadow  Port=5
  desLaneA4 : InportShadow
  desLaneA5 : InportShadow  Port=3
  desLaneA6 : InportShadow  Port=4
  PlanX : Outport
  PlanY : Outport  Port=2
  PlanTheta : Outport  Port=3
  idx : Outport  Port=4
  PreviewX : Outport  Port=5
  PreviewY : Outport  Port=6
  PreviewTheta : Outport  Port=7
  numTraj : Outport  Port=8
  ref_curvature : Outport  Port=9
  lateral_error : Outport  Port=10
  lateral_error_rate : Outport  Port=11
  heading_error : Outport  Port=12
  heading_error_rate : Outport  Port=13
  wires:
  desLaneA6/1 -> Subsystem/6(LCS_IN_desLaneA3)
  desLaneA5/1 -> Subsystem/5(LCS_IN_desLaneA2)
  desLaneA4/1 -> Subsystem/4(LCS_IN_desLaneA0)
  Veh_Speed_kph/1 -> Subsystem/2(Spd_kph)
  Veh_Speed_ms1/1 -> Subsystem/3(VehSpd_ms)
  TarDangerLevel/1 -> Subsystem/1(TarDangerLevel), FrenetTrajectory/7(TarDangerlLevel)
  Subsystem/2(AyDtLimit) -> FrenetTrajectory/9(AyDtLimit)
  Subsystem/1(Preview_T) -> FrenetTrajectory/8(PreView_T)
  Long_Acc/1 -> FrenetTrajectory/11(axEgo)
  FrenetTrajectory/13(heading_error_rate) -> heading_error_rate/1
  FrenetTrajectory/12(heading_error) -> heading_error/1
  FrenetTrajectory/11(lateral_error_rate) -> lateral_error_rate/1
  FrenetTrajectory/10(lateral_error) -> lateral_error/1
  FrenetTrajectory/9(ref_curvature) -> ref_curvature/1
  FrenetTrajectory/8(numTraj) -> numTraj/1
  FrenetTrajectory/7(PreviewTheta) -> PreviewTheta/1
  FrenetTrajectory/6(PreviewY) -> PreviewY/1
  FrenetTrajectory/5(PreviewX) -> PreviewX/1
  FrenetTrajectory/4(idx) -> idx/1
  FrenetTrajectory/3(PlanTheta) -> PlanTheta/1
  FrenetTrajectory/2(PlanY) -> PlanY/1
  FrenetTrajectory/1(PlanX) -> PlanX/1
  YawRate/1 -> FrenetTrajectory/6(YawRate)
  Veh_Speed_ms/1 -> FrenetTrajectory/5(Veh_Speed)
  desLaneA3/1 -> FrenetTrajectory/4(A3)
  desLaneA2/1 -> FrenetTrajectory/3(A2)
  desLaneA1/1 -> FrenetTrajectory/2(A1)
  desLaneA0/1 -> FrenetTrajectory/1(A0)
  kapEgo/1 -> FrenetTrajectory/12(kapEgo)
  Subsystem/3(Min_Plan_Dis) -> FrenetTrajectory/10(Min_Plan_Dis)

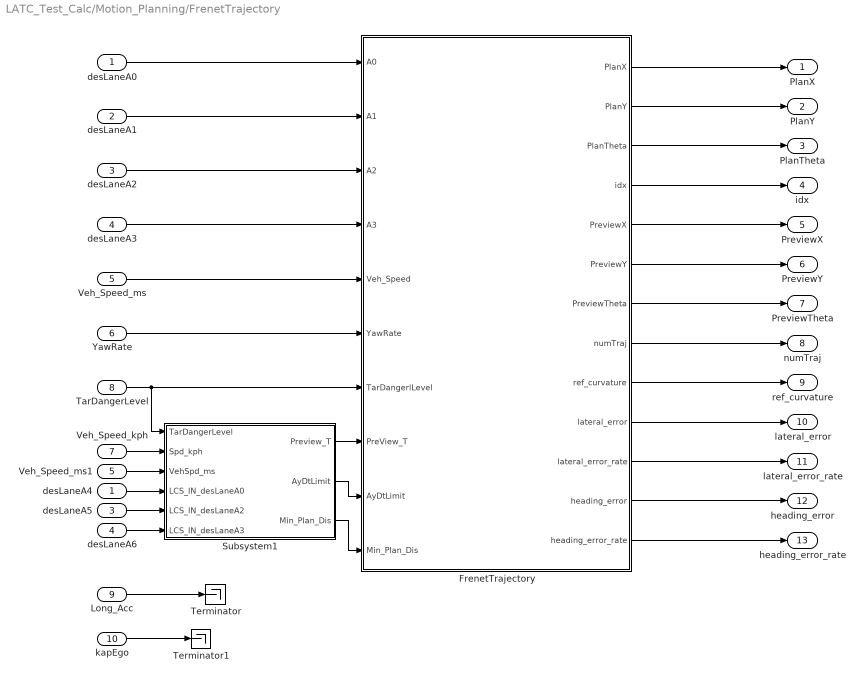
== system LATC_Test_Calc/Motion_Planning/FrenetTrajectory ==
  desLaneA0 : Inport
  desLaneA1 : Inport  Port=2
  desLaneA2 : Inport  Port=3
  desLaneA3 : Inport  Port=4
  Veh_Speed_ms : Inport  Port=5
  YawRate : Inport  Port=6
  Veh_Speed_kph : Inport  Port=7
  TarDangerLevel : Inport  Port=8
  Long_Acc : Inport  Port=9
  kapEgo : Inport  Port=10
  FrenetTrajectory : MATLAB Function  TreatAsAtomicUnit=on
  Subsystem1 : Subsystem
  Terminator : Terminator
  Terminator1 : Terminator
  Veh_Speed_ms1 : InportShadow  Port=5
  desLaneA4 : InportShadow
  desLaneA5 : InportShadow  Port=3
  desLaneA6 : InportShadow  Port=4
  PlanX : Outport
  PlanY : Outport  Port=2
  PlanTheta : Outport  Port=3
  idx : Outport  Port=4
  PreviewX : Outport  Port=5
  PreviewY : Outport  Port=6
  PreviewTheta : Outport  Port=7
  numTraj : Outport  Port=8
  ref_curvature : Outport  Port=9
  lateral_error : Outport  Port=10
  lateral_error_rate : Outport  Port=11
  heading_error : Outport  Port=12
  heading_error_rate : Outport  Port=13
  wires:
  desLaneA0/1 -> FrenetTrajectory/1(A0)
  desLaneA1/1 -> FrenetTrajectory/2(A1)
  desLaneA2/1 -> FrenetTrajectory/3(A2)
  desLaneA3/1 -> FrenetTrajectory/4(A3)
  Veh_Speed_ms/1 -> FrenetTrajectory/5(Veh_Speed)
  YawRate/1 -> FrenetTrajectory/6(YawRate)
  FrenetTrajectory/1(PlanX) -> PlanX/1
  FrenetTrajectory/2(PlanY) -> PlanY/1
  FrenetTrajectory/3(PlanTheta) -> PlanTheta/1
  FrenetTrajectory/4(idx) -> idx/1
  FrenetTrajectory/5(PreviewX) -> PreviewX/1
  FrenetTrajectory/6(PreviewY) -> PreviewY/1
  FrenetTrajectory/7(PreviewTheta) -> PreviewTheta/1
  FrenetTrajectory/8(numTraj) -> numTraj/1
  FrenetTrajectory/9(ref_curvature) -> ref_curvature/1
  FrenetTrajectory/10(lateral_error) -> lateral_error/1
  FrenetTrajectory/11(lateral_error_rate) -> lateral_error_rate/1
  FrenetTrajectory/12(heading_error) -> heading_error/1
  FrenetTrajectory/13(heading_error_rate) -> heading_error_rate/1
  Long_Acc/1 -> Terminator/1
  Subsystem1/1(Preview_T) -> FrenetTrajectory/8(PreView_T)
  Subsystem1/2(AyDtLimit) -> FrenetTrajectory/9(AyDtLimit)
  TarDangerLevel/1 -> Subsystem1/1(TarDangerLevel), FrenetTrajectory/7(TarDangerlLevel)
  Veh_Speed_ms1/1 -> Subsystem1/3(VehSpd_ms)
  Veh_Speed_kph/1 -> Subsystem1/2(Spd_kph)
  desLaneA4/1 -> Subsystem1/4(LCS_IN_desLaneA0)
  desLaneA5/1 -> Subsystem1/5(LCS_IN_desLaneA2)
  desLaneA6/1 -> Subsystem1/6(LCS_IN_desLaneA3)
  kapEgo/1 -> Terminator1/1
  Subsystem1/3(Min_Plan_Dis) -> FrenetTrajectory/10(Min_Plan_Dis)

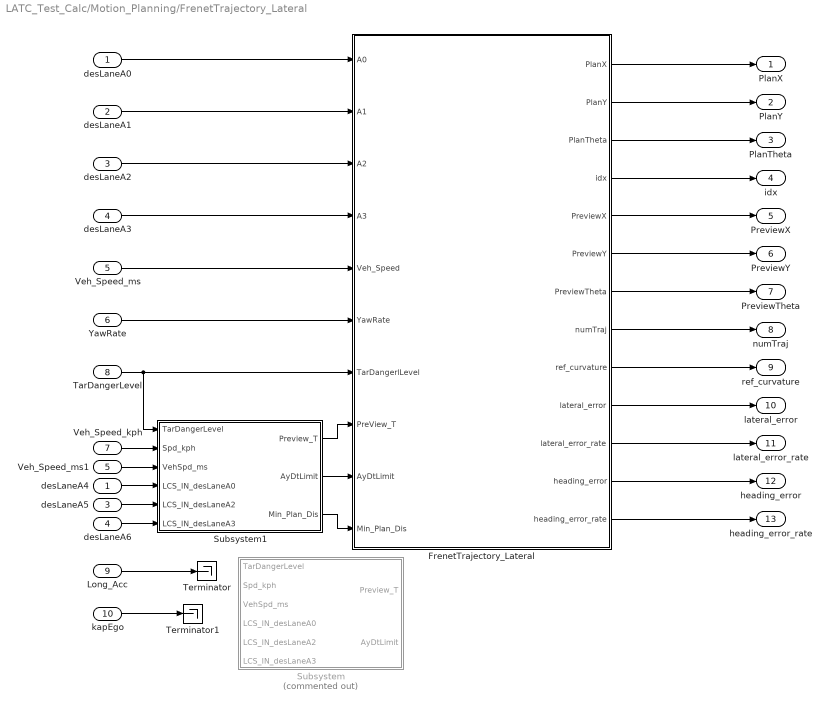
== system LATC_Test_Calc/Motion_Planning/FrenetTrajectory_Lateral ==
  desLaneA0 : Inport
  desLaneA1 : Inport  Port=2
  desLaneA2 : Inport  Port=3
  desLaneA3 : Inport  Port=4
  Veh_Speed_ms : Inport  Port=5
  YawRate : Inport  Port=6
  Veh_Speed_kph : Inport  Port=7
  TarDangerLevel : Inport  Port=8
  Long_Acc : Inport  Port=9
  kapEgo : Inport  Port=10
  FrenetTrajectory_Lateral : MATLAB Function  TreatAsAtomicUnit=on
  Subsystem : Subsystem  Commented=on
  Subsystem1 : Subsystem
  Terminator : Terminator
  Terminator1 : Terminator
  Veh_Speed_ms1 : InportShadow  Port=5
  desLaneA4 : InportShadow
  desLaneA5 : InportShadow  Port=3
  desLaneA6 : InportShadow  Port=4
  PlanX : Outport
  PlanY : Outport  Port=2
  PlanTheta : Outport  Port=3
  idx : Outport  Port=4
  PreviewX : Outport  Port=5
  PreviewY : Outport  Port=6
  PreviewTheta : Outport  Port=7
  numTraj : Outport  Port=8
  ref_curvature : Outport  Port=9
  lateral_error : Outport  Port=10
  lateral_error_rate : Outport  Port=11
  heading_error : Outport  Port=12
  heading_error_rate : Outport  Port=13
  wires:
  desLaneA4/1 -> Subsystem1/4(LCS_IN_desLaneA0)
  Veh_Speed_kph/1 -> Subsystem1/2(Spd_kph)
  Veh_Speed_ms1/1 -> Subsystem1/3(VehSpd_ms)
  TarDangerLevel/1 -> Subsystem1/1(TarDangerLevel), FrenetTrajectory_Lateral/7(TarDangerlLevel)
  Subsystem1/2(AyDtLimit) -> FrenetTrajectory_Lateral/9(AyDtLimit)
  Subsystem1/1(Preview_T) -> FrenetTrajectory_Lateral/8(PreView_T)
  Long_Acc/1 -> Terminator/1
  FrenetTrajectory_Lateral/13(heading_error_rate) -> heading_error_rate/1
  FrenetTrajectory_Lateral/12(heading_error) -> heading_error/1
  FrenetTrajectory_Lateral/11(lateral_error_rate) -> lateral_error_rate/1
  FrenetTrajectory_Lateral/10(lateral_error) -> lateral_error/1
  FrenetTrajectory_Lateral/9(ref_curvature) -> ref_curvature/1
  FrenetTrajectory_Lateral/8(numTraj) -> numTraj/1
  FrenetTrajectory_Lateral/7(PreviewTheta) -> PreviewTheta/1
  FrenetTrajectory_Lateral/6(PreviewY) -> PreviewY/1
  FrenetTrajectory_Lateral/5(PreviewX) -> PreviewX/1
  FrenetTrajectory_Lateral/4(idx) -> idx/1
  FrenetTrajectory_Lateral/3(PlanTheta) -> PlanTheta/1
  FrenetTrajectory_Lateral/2(PlanY) -> PlanY/1
  FrenetTrajectory_Lateral/1(PlanX) -> PlanX/1
  YawRate/1 -> FrenetTrajectory_Lateral/6(YawRate)
  Veh_Speed_ms/1 -> FrenetTrajectory_Lateral/5(Veh_Speed)
  desLaneA3/1 -> FrenetTrajectory_Lateral/4(A3)
  desLaneA2/1 -> FrenetTrajectory_Lateral/3(A2)
  desLaneA1/1 -> FrenetTrajectory_Lateral/2(A1)
  desLaneA0/1 -> FrenetTrajectory_Lateral/1(A0)
  desLaneA5/1 -> Subsystem1/5(LCS_IN_desLaneA2)
  desLaneA6/1 -> Subsystem1/6(LCS_IN_desLaneA3)
  kapEgo/1 -> Terminator1/1
  Subsystem1/3(Min_Plan_Dis) -> FrenetTrajectory_Lateral/10(Min_Plan_Dis)

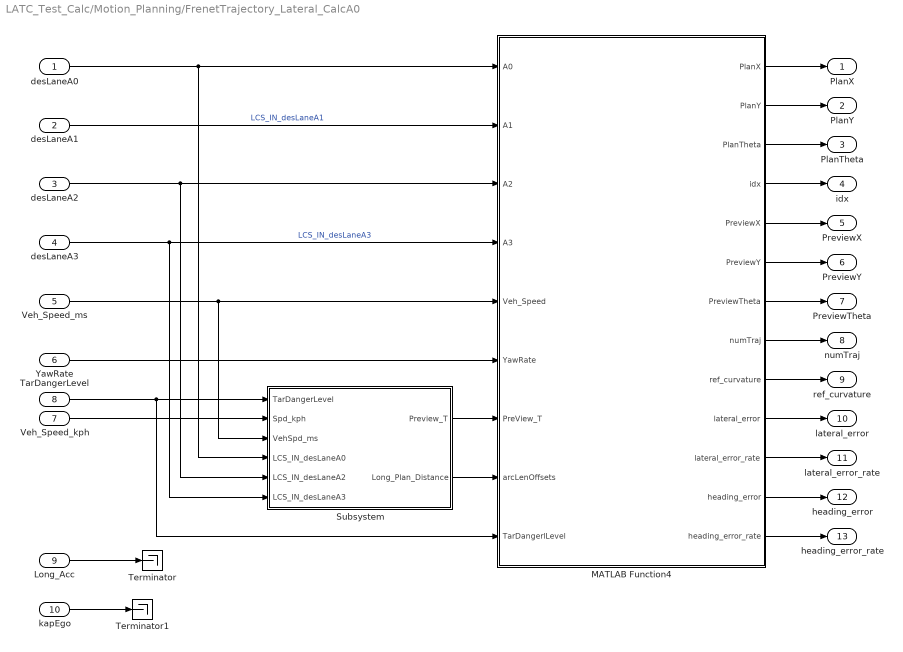
== system LATC_Test_Calc/Motion_Planning/FrenetTrajectory_Lateral_CalcA0 ==
  desLaneA0 : Inport
  desLaneA1 : Inport  Port=2
  desLaneA2 : Inport  Port=3
  desLaneA3 : Inport  Port=4
  Veh_Speed_ms : Inport  Port=5
  YawRate : Inport  Port=6
  Veh_Speed_kph : Inport  Port=7
  TarDangerLevel : Inport  Port=8
  Long_Acc : Inport  Port=9
  kapEgo : Inport  Port=10
  MATLAB Function4 : MATLAB Function  TreatAsAtomicUnit=on
  Subsystem : Subsystem
  Terminator : Terminator
  Terminator1 : Terminator
  PlanX : Outport
  PlanY : Outport  Port=2
  PlanTheta : Outport  Port=3
  idx : Outport  Port=4
  PreviewX : Outport  Port=5
  PreviewY : Outport  Port=6
  PreviewTheta : Outport  Port=7
  numTraj : Outport  Port=8
  ref_curvature : Outport  Port=9
  lateral_error : Outport  Port=10
  lateral_error_rate : Outport  Port=11
  heading_error : Outport  Port=12
  heading_error_rate : Outport  Port=13
  wires:
  desLaneA0/1 -> Subsystem/4(LCS_IN_desLaneA0), MATLAB Function4/1(A0)
  desLaneA3/1 -> Subsystem/6(LCS_IN_desLaneA3), MATLAB Function4/4(A3)  "LCS_IN_desLaneA3"
  Veh_Speed_kph/1 -> Subsystem/2(Spd_kph)
  Veh_Speed_ms/1 -> Subsystem/3(VehSpd_ms), MATLAB Function4/5(Veh_Speed)
  Subsystem/2(Long_Plan_Distance) -> MATLAB Function4/8(arcLenOffsets)
  YawRate/1 -> MATLAB Function4/6(YawRate)
  TarDangerLevel/1 -> MATLAB Function4/9(TarDangerlLevel), Subsystem/1(TarDangerLevel)
  Subsystem/1(Preview_T) -> MATLAB Function4/7(PreView_T)
  desLaneA2/1 -> Subsystem/5(LCS_IN_desLaneA2), MATLAB Function4/3(A2)
  desLaneA1/1 -> MATLAB Function4/2(A1)  "LCS_IN_desLaneA1"
  Long_Acc/1 -> Terminator/1
  MATLAB Function4/1(PlanX) -> PlanX/1
  MATLAB Function4/2(PlanY) -> PlanY/1
  MATLAB Function4/13(heading_error_rate) -> heading_error_rate/1
  MATLAB Function4/12(heading_error) -> heading_error/1
  MATLAB Function4/11(lateral_error_rate) -> lateral_error_rate/1
  MATLAB Function4/10(lateral_error) -> lateral_error/1
  MATLAB Function4/9(ref_curvature) -> ref_curvature/1
  MATLAB Function4/8(numTraj) -> numTraj/1
  MATLAB Function4/7(PreviewTheta) -> PreviewTheta/1
  MATLAB Function4/6(PreviewY) -> PreviewY/1
  MATLAB Function4/5(PreviewX) -> PreviewX/1
  MATLAB Function4/4(idx) -> idx/1
  MATLAB Function4/3(PlanTheta) -> PlanTheta/1
  kapEgo/1 -> Terminator1/1

== system LATC_Test_Calc/SteerAngSlopeCalc/Switch Case Action Subsystem ==
  Flg : Inport
  StateHoldTime : Inport  Port=2
  Action Port : ActionPort  ActionPortLabel=case [ 1 2 3 4 5 ]:
  LC_start_slope : Lookup_n-D  BreakpointsForDimension1=P_LCS_StateActiveFlg_BP  BreakpointsForDimension2=P_LCS_StateActive_HoldTime_BP  Table=P_LCS_StateActiv_AngleSlope  ExtrapMethod=Clip  UseLastTableValue=on  InternalRulePriority=Speed  OutDataTypeStr=single  RndMeth=Simplest
      settings: InputPortMap=u0,u1
  Out1 : Outport
  wires:
  StateHoldTime/1 -> LC_start_slope/2
  LC_start_slope/1 -> Out1/1
  Flg/1 -> LC_start_slope/1

== system LATC_Test_Calc/SteerAngSlopeCalc/Switch Case Action Subsystem1 ==
  Action Port : ActionPort  ActionPortLabel=default:
  Constant : Constant  Value=100  OutDataTypeStr=single
  Out1 : Outport
  wires:
  Constant/1 -> Out1/1

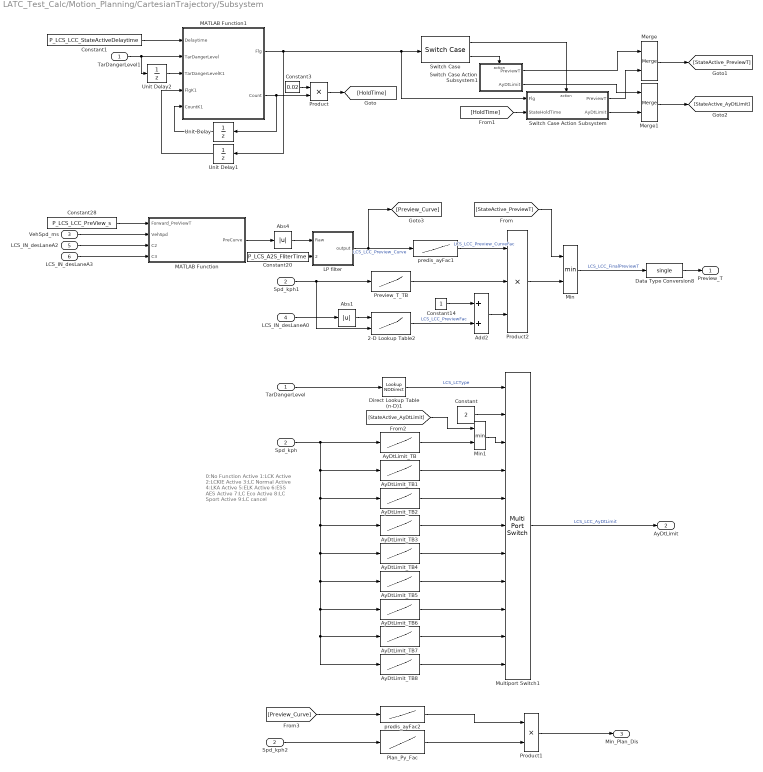
== system LATC_Test_Calc/Motion_Planning/CartesianTrajectory/Subsystem ==
  note: 0:No Function Active
      | 1:LCK Active
      | 2:LCKIE Active
      | 3:LC Normal Active
      | 4:LKA Active
      | 5:ELK Active
      | 6:ESS AES Active
      | 7:LC Eco Active
      | 8:LC Sport Active
      | 9:LC cancel
  TarDangerLevel : Inport
  Spd_kph : Inport  Port=2
  VehSpd_ms : Inport  Port=3
  LCS_IN_desLaneA0 : Inport  Port=4
  LCS_IN_desLaneA2 : Inport  Port=5
  LCS_IN_desLaneA3 : Inport  Port=6
  2-D Lookup Table2 : Lookup_n-D  BreakpointsForDimension1=P_LCS_A0_Dis_BP  BreakpointsForDimension2=P_LCS_preDis_spd  Table=P_LCS_LCC_PreView_Fac  ExtrapMethod=Clip  UseLastTableValue=on  InternalRulePriority=Speed  RndMeth=Simplest  InputSameDT=on
      settings: InputPortMap=u0,u1
  Abs1 : Abs
  Abs4 : Abs
  Add2 : Sum
  AyDtLimit_TB : Lookup_n-D  NumberOfTableDimensions=1  BreakpointsForDimension1=P_LCS_preDis_spd  Table=P_LCS_LCC_LCK_AyDtLimit_TBL  ExtrapMethod=Clip  UseLastTableValue=on  InternalRulePriority=Speed  RndMeth=Simplest  InputSameDT=on
  AyDtLimit_TB1 : Lookup_n-D  NumberOfTableDimensions=1  BreakpointsForDimension1=P_LCS_preDis_spd  Table=P_LCS_LCC_LCK_AyDtLimit_TBL  ExtrapMethod=Clip  UseLastTableValue=on  InternalRulePriority=Speed  RndMeth=Simplest  InputSameDT=on
  AyDtLimit_TB2 : Lookup_n-D  NumberOfTableDimensions=1  BreakpointsForDimension1=P_LCS_preDis_spd  Table=P_LCS_LCC_LC_Normal_AyDtLimit_TBL  ExtrapMethod=Clip  UseLastTableValue=on  InternalRulePriority=Speed  RndMeth=Simplest  InputSameDT=on
  AyDtLimit_TB3 : Lookup_n-D  NumberOfTableDimensions=1  BreakpointsForDimension1=P_LCS_preDis_spd  Table=P_LCS_LCC_LKA_AyDtLimit_TBL  ExtrapMethod=Clip  UseLastTableValue=on  InternalRulePriority=Speed  RndMeth=Simplest  InputSameDT=on
  AyDtLimit_TB4 : Lookup_n-D  NumberOfTableDimensions=1  BreakpointsForDimension1=P_LCS_preDis_spd  Table=P_LCS_LCC_ELK_AyDtLimit_TBL  ExtrapMethod=Clip  UseLastTableValue=on  InternalRulePriority=Speed  RndMeth=Simplest  InputSameDT=on
  AyDtLimit_TB5 : Lookup_n-D  NumberOfTableDimensions=1  BreakpointsForDimension1=P_LCS_preDis_spd  Table=P_LCS_LCC_ESS_AyDtLimit_TBL  ExtrapMethod=Clip  UseLastTableValue=on  InternalRulePriority=Speed  RndMeth=Simplest  InputSameDT=on
  AyDtLimit_TB6 : Lookup_n-D  NumberOfTableDimensions=1  BreakpointsForDimension1=P_LCS_preDis_spd  Table=P_LCS_LCC_Eco_AyDtLimit_TBL  ExtrapMethod=Clip  UseLastTableValue=on  InternalRulePriority=Speed  RndMeth=Simplest  InputSameDT=on
  AyDtLimit_TB7 : Lookup_n-D  NumberOfTableDimensions=1  BreakpointsForDimension1=P_LCS_preDis_spd  Table=P_LCS_LCC_Sport_AyDtLimit_TBL  ExtrapMethod=Clip  UseLastTableValue=on  InternalRulePriority=Speed  RndMeth=Simplest  InputSameDT=on
  AyDtLimit_TB8 : Lookup_n-D  NumberOfTableDimensions=1  BreakpointsForDimension1=P_LCS_preDis_spd  Table=P_LCS_LCC_LC_AyDtLimit_TBL  ExtrapMethod=Clip  UseLastTableValue=on  InternalRulePriority=Speed  RndMeth=Simplest  InputSameDT=on
  Constant : Constant  Value=2  OutDataTypeStr=single
  Constant1 : Constant  Value=P_LCS_LCC_StateActiveDelaytime  OutDataTypeStr=uint16
  Constant14 : Constant  OutDataTypeStr=single
  Constant20 : Constant  Value=P_LCS_A2S_FliterTime
  Constant28 : Constant  Value=P_LCS_LCC_PreView_s  OutDataTypeStr=single
  Constant3 : Constant  Value=0.02
  Data Type Conversion8 : DataTypeConversion  OutDataTypeStr=single
  Direct Lookup Table (n-D)1 : LookupNDDirect  NumberOfTableDimensions=1  Table=[0 1 2 3 4 5 6 7 8 9]  TableDataTypeStr=uint8
  LP filter : Subsystem
  MATLAB Function : MATLAB Function  TreatAsAtomicUnit=on
  MATLAB Function1 : MATLAB Function  TreatAsAtomicUnit=on
  Merge : Merge
  Merge1 : Merge
  Min : MinMax  Inputs=2
  Min1 : MinMax  Inputs=2
  Multiport Switch1 : MultiPortSwitch  DataPortOrder=Zero-based contiguous  Inputs=10  zeroidx=on
  Plan_Py_Fac : Lookup_n-D  NumberOfTableDimensions=1  BreakpointsForDimension1=P_LCS_DeltaEps_SpdBp  Table=P_LCS_LCC_Min_Plan_Dis  ExtrapMethod=Clip  UseLastTableValue=on  InternalRulePriority=Speed  RndMeth=Simplest  InputSameDT=on
  Preview_T_TB : Lookup_n-D  NumberOfTableDimensions=1  BreakpointsForDimension1=P_LCS_preDis_spd  Table=P_LCS_LCC_PreViewT  ExtrapMethod=Clip  UseLastTableValue=on  InternalRulePriority=Speed  RndMeth=Simplest  InputSameDT=on
  Product : Product
  Product1 : Product
  Product2 : Product  Inputs=3
  Spd_kph1 : InportShadow  Port=2
  Spd_kph2 : InportShadow  Port=2
  Switch Case : SwitchCase  CaseConditions={[1]}
  Switch Case Action Subsystem : Subsystem  TreatAsAtomicUnit=on
  Switch Case Action Subsystem1 : Subsystem  TreatAsAtomicUnit=on
  TarDangerLevel1 : InportShadow
  Unit Delay : UnitDelay  SampleTime=-1  HasFrameUpgradeWarning=on
  Unit Delay1 : UnitDelay  SampleTime=-1  HasFrameUpgradeWarning=on
  Unit Delay2 : UnitDelay  SampleTime=-1  HasFrameUpgradeWarning=on
  predis_ayFac1 : Lookup_n-D  NumberOfTableDimensions=1  BreakpointsForDimension1=P_LCS_A2_Curve_BP  Table=P_LCS_LCC_PreViewCurve_Fac  ExtrapMethod=Clip  UseLastTableValue=on  InternalRulePriority=Speed  RndMeth=Simplest  InputSameDT=on
  predis_ayFac2 : Lookup_n-D  NumberOfTableDimensions=1  BreakpointsForDimension1=P_LCS_A2_Curve_BP  Table=P_LCS_LCC_PreCur_Min_Plan_Dis_Fac  ExtrapMethod=Clip  UseLastTableValue=on  InternalRulePriority=Speed  RndMeth=Simplest  InputSameDT=on
  Preview_T : Outport  OutDataTypeStr=single
  AyDtLimit : Outport  Port=2  OutDataTypeStr=single
  Min_Plan_Dis : Outport  Port=3  OutDataTypeStr=single
  wires:
  Min1/1 -> Multiport Switch1/3
  [StateActive_AyDtLimit] -> Min1/1
  Product2/1 -> Min/2
  [StateActive_PreviewT] -> Min/1
  Merge1/1 -> [StateActive_AyDtLimit]
  Merge/1 -> [StateActive_PreviewT]
  Switch Case Action Subsystem1/2(AyDtLimit) -> Merge1/1
  Switch Case Action Subsystem/2(AyDtLimit) -> Merge1/2
  Product/1 -> [HoldTime]
  [HoldTime] -> Switch Case Action Subsystem/2(StateHoldTime)
  Constant3/1 -> Product/1
  Switch Case/2 -> Switch Case Action Subsystem1/Action
  MATLAB Function1/2(Count) -> Unit Delay/1, Product/2
  Switch Case Action Subsystem/1(PreviewT) -> Merge/2
  Switch Case/1 -> Switch Case Action Subsystem/Action
  Switch Case Action Subsystem1/1(PreviewT) -> Merge/1
  MATLAB Function1/1(Flg) -> Switch Case/1, Switch Case Action Subsystem/1(Flg), Unit Delay1/1
  Constant1/1 -> MATLAB Function1/1(Delaytime)
  Unit Delay2/1 -> MATLAB Function1/3(TarDangerLevelK1)
  TarDangerLevel1/1 -> MATLAB Function1/2(TarDangerLevel), Unit Delay2/1
  Unit Delay1/1 -> MATLAB Function1/4(FlgK1)
  Unit Delay/1 -> MATLAB Function1/5(CountK1)
  AyDtLimit_TB8/1 -> Multiport Switch1/11
  AyDtLimit_TB7/1 -> Multiport Switch1/10
  AyDtLimit_TB6/1 -> Multiport Switch1/9
  AyDtLimit_TB5/1 -> Multiport Switch1/8
  AyDtLimit_TB4/1 -> Multiport Switch1/7
  AyDtLimit_TB3/1 -> Multiport Switch1/6
  AyDtLimit_TB2/1 -> Multiport Switch1/5
  AyDtLimit_TB1/1 -> Multiport Switch1/4
  Constant/1 -> Multiport Switch1/2
  Constant28/1 -> MATLAB Function/1(Forward_PreViewT)
  predis_ayFac1/1 -> Product2/1  "LCS_LCC_Preview_CurveFac"
  LP filter/1(output) -> [Preview_Curve], predis_ayFac1/1  "LCS_LCC_Preview_Curve"
  Constant20/1 -> LP filter/2(TorqFilterTime)
  Abs4/1 -> LP filter/1(Raw)
  MATLAB Function/1(PreCurve) -> Abs4/1
  LCS_IN_desLaneA3/1 -> MATLAB Function/4(C3)
  LCS_IN_desLaneA2/1 -> MATLAB Function/3(C2)
  VehSpd_ms/1 -> MATLAB Function/2(VehSpd)
  Data Type Conversion8/1 -> Preview_T/1
  Min/1 -> Data Type Conversion8/1  "LCS_LCC_FinalPreviewT"
  LCS_IN_desLaneA0/1 -> Abs1/1
  Abs1/1 -> 2-D Lookup Table2/1
  Spd_kph1/1 -> Preview_T_TB/1, 2-D Lookup Table2/2
  Add2/1 -> Product2/3
  Constant14/1 -> Add2/1
  2-D Lookup Table2/1 -> Add2/2  "LCS_LCC_PreviewFac"
  Preview_T_TB/1 -> Product2/2
  AyDtLimit_TB/1 -> Min1/2
  Multiport Switch1/1 -> AyDtLimit/1  "LCS_LCC_AyDtLimit"
  Spd_kph/1 -> AyDtLimit_TB/1, AyDtLimit_TB1/1, AyDtLimit_TB2/1, AyDtLimit_TB4/1, AyDtLimit_TB5/1, AyDtLimit_TB7/1, AyDtLimit_TB8/1, AyDtLimit_TB6/1, AyDtLimit_TB3/1
  TarDangerLevel/1 -> Direct Lookup Table (n-D)1/1
  Direct Lookup Table (n-D)1/1 -> Multiport Switch1/1  "LCS_LCType"
  Plan_Py_Fac/1 -> Product1/2
  Spd_kph2/1 -> Plan_Py_Fac/1
  [Preview_Curve] -> predis_ayFac2/1
  Product1/1 -> Min_Plan_Dis/1
  predis_ayFac2/1 -> Product1/1
